simulink model "Simulink_File"  (R2021a)
settings: Solver=VariableStepAuto  StartTime=0.0  StopTime=10.0  RelTol=1e-3
undefined symbols (not defined in the file or in its folder): A, B, C, D, x0
libraries: vrlib x2, aerolibanimutils x1
settings Model: Creator=J44381  LastModifiedBy=vicen
settings SolverCC: AlgebraicLoopSolver=TrustRegion
settings DebuggingCC: SFMachineParentedDataDiag=warning

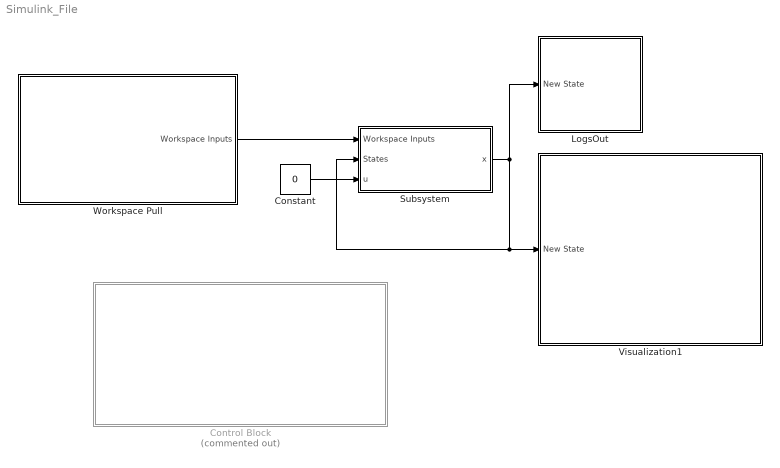
== system Simulink_File ==
  Constant : Constant  Value=0
  Control Block : Subsystem  Commented=on
  LogsOut : Subsystem
  Subsystem : Subsystem
  Visualization1 : Subsystem
  Workspace Pull : Subsystem
  wires:
  Workspace Pull/1("Workspace Inputs ") -> Subsystem/1("Workspace Inputs ")
  Subsystem/1(x) -> LogsOut/1(New State), Visualization1/1(New State), Subsystem/2(States)
  Constant/1 -> Subsystem/3(u)

== system Simulink_File/Control Block ==

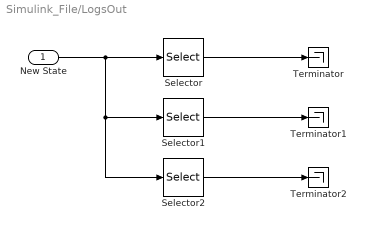
== system Simulink_File/LogsOut ==
  New State : Inport
  Selector : Selector  InputPortWidth=6  IndexOptions=Index vector (dialog)  Indices=1  OutputSizes=1
  Selector1 : Selector  InputPortWidth=6  IndexOptions=Index vector (dialog)  Indices=2  OutputSizes=1
  Selector2 : Selector  InputPortWidth=6  IndexOptions=Index vector (dialog)  Indices=3  OutputSizes=1
  Terminator : Terminator
  Terminator1 : Terminator
  Terminator2 : Terminator
  wires:
  Selector/1 -> Terminator/1
  Selector1/1 -> Terminator1/1
  Selector2/1 -> Terminator2/1
  New State/1 -> Selector2/1, Selector1/1, Selector/1

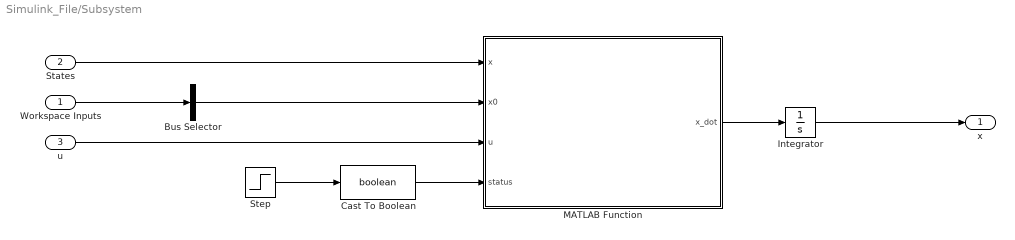
== system Simulink_File/Subsystem ==
  "Workspace Inputs " : Inport
  States : Inport  Port=2
  u : Inport  Port=3
  Bus Selector : BusSelector  OutputSignals=Initial States  OutputAsBus=on
  Cast To Boolean : DataTypeConversion  OutDataTypeStr=boolean
  Integrator : Integrator  InitialCondition=[x0.x;x0.theta1;x0.theta2;x0.x_dot;x0.theta1_dot;x0.theta2_dot]
  MATLAB Function : MATLAB Function  TreatAsAtomicUnit=on
  Step : Step  SampleTime=0
  x : Outport
  wires:
  MATLAB Function/1(x_dot) -> Integrator/1
  States/1 -> MATLAB Function/1(x)
  "Workspace Inputs "/1 -> Bus Selector/1
  u/1 -> MATLAB Function/3(u)
  Bus Selector/1 -> MATLAB Function/2(x0)
  Integrator/1 -> x/1
  Step/1 -> Cast To Boolean/1
  Cast To Boolean/1 -> MATLAB Function/4(status)

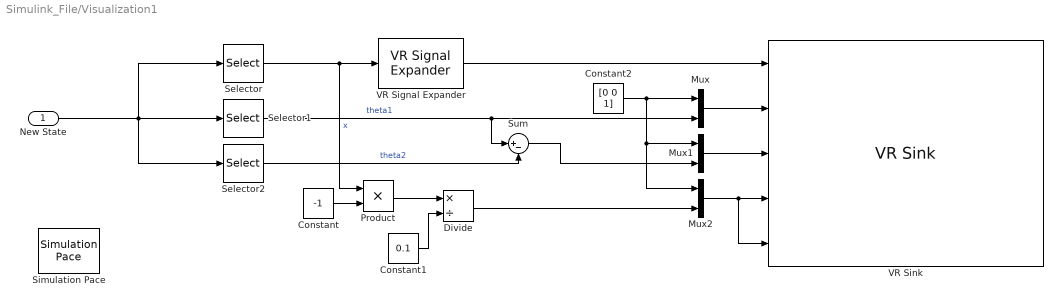
== system Simulink_File/Visualization1 ==
  New State : Inport
  Constant : Constant  Value=-1
  Constant1 : Constant  Value=0.1
  Constant2 : Constant  Value=[0 0 1]
  Divide : Product  Inputs=*/
  Mux : Mux  Inputs=2
  Mux1 : Mux  Inputs=2
  Mux2 : Mux  Inputs=2
  Product : Product
  Selector : Selector  InputPortWidth=6  IndexOptions=Index vector (dialog)  Indices=1  OutputSizes=1
  Selector1 : Selector  InputPortWidth=6  IndexOptions=Index vector (dialog)  Indices=2  OutputSizes=1
  Selector2 : Selector  InputPortWidth=6  IndexOptions=Index vector (dialog)  Indices=3  OutputSizes=1
  Simulation Pace : aerolibanimutils/Simulation Pace  SimulationPace=1  SleepMode=Auto  OutputPaceError=off  SampleTime=1/30
  Sum : Sum  Inputs=|+-
  VR Signal Expander : vrlib/VR Signal Expander  outwidth=3  outidx=[1]
  VR Sink : vrlib/VR Sink  InstantiateOnLoad=on  SampleTime=0.1  ViewEnable=on  RemoteChange=off  RemoteView=off  FieldsWritten=Cart.translation.3.1.1.double#Rotation1.rotation.4.1.1.double#Rotation2.rotation.4.1.1.double#Axis_Rotate.rotation.4.1.1.double#Axis_Rotate2.rotation.4.1.1.double  WorldFileName=Cart_Actual.WRL  AutoView=off  VideoDimensions=[]  AllowVariableSize=off
  wires:
  New State/1 -> Selector/1, Selector2/1, Selector1/1
  Selector/1 -> VR Signal Expander/1, Product/1  "x"
  Selector1/1 -> Sum/1, Mux/2  "theta1"
  Product/1 -> Divide/1
  Constant/1 -> Product/2
  Constant1/1 -> Divide/2
  Constant2/1 -> Mux1/1, Mux2/1, Mux/1
  Selector2/1 -> Sum/2  "theta2"
  Divide/1 -> Mux2/2
  Sum/1 -> Mux1/2
  VR Signal Expander/1 -> VR Sink/1
  Mux/1 -> VR Sink/2
  Mux1/1 -> VR Sink/3
  Mux2/1 -> VR Sink/4, VR Sink/5

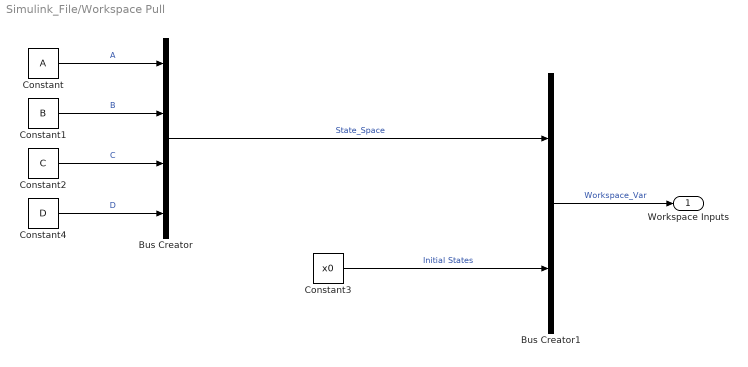
== system Simulink_File/Workspace Pull ==
  Bus Creator : BusCreator  Inputs=4
  Bus Creator1 : BusCreator  Inputs=2
  Constant : Constant  Value=A  VectorParams1D=off
  Constant1 : Constant  Value=B  VectorParams1D=off
  Constant2 : Constant  Value=C  VectorParams1D=off
  Constant3 : Constant  Value=x0  VectorParams1D=off  OutDataTypeStr=Bus: State_bus
  Constant4 : Constant  Value=D  VectorParams1D=off
  "Workspace Inputs " : Outport
  wires:
  Constant/1 -> Bus Creator/1  "A"
  Constant1/1 -> Bus Creator/2  "B"
  Constant2/1 -> Bus Creator/3  "C"
  Constant4/1 -> Bus Creator/4  "D"
  Bus Creator/1 -> Bus Creator1/1  "State_Space"
  Bus Creator1/1 -> "Workspace Inputs "/1  "Workspace_Var"
  Constant3/1 -> Bus Creator1/2  "Initial States"

== matlab function Simulink_File/Subsystem/MATLAB Function ==
  data: x input; x0 input; u input; x_dot output; status input
function x_dot  = Nonlinear_Dynamics(x,x0,u,status)
    if status == false
        x2 = x0.theta1;
        x3 = x0.theta2;
        x4 = x0.x_dot;
        x5 = x0.theta1_dot;
        x6 = x0.theta2_dot;
        u1 = u;
    else
        x2 = x(2);
        x3 = x(3);
        x4 = x(4);
        x5 = x(5);
        x6 = x(6);
        u1 = u;
    end
    % Insert Equations
    x_dot = double([
       x4;
       x5;
       x6;
       x5*((15*x5*sin(x2 - x3)*(cos(x3) - cos(x2 - x3)*cos(x2)))/(2*(25*cos(x2)^2 + 15*cos(x3)^2 + 33*cos(x2 - x3)^2 - 30*cos(x2 - x3)*cos(x2)*cos(x3) - 55)) + (5*x5*sin(x2)*(3*cos(x2 - x3)^2 - 5))/(2*(25*cos(x2)^2 + 15*cos(x3)^2 + 33*cos(x2 - x3)^2 - 30*cos(x2 - x3)*cos(x2)*cos(x3) - 55))) - x6*((9*x6*sin(x2 - x3)*(5*cos(x2) - 3*cos(x2 - x3)*cos(x3)))/(4*(25*cos(x2)^2 + 15*cos(x3)^2 + 33*cos(x2 - x3)^2 - 30*cos(x2 - x3)*cos(x2)*cos(x3) - 55)) - (9*x6*sin(x3)*(3*cos(x2 - x3)^2 - 5))/(4*(25*cos(x2)^2 + 15*cos(x3)^2 + 33*cos(x2 - x3)^2 - 30*cos(x2 - x3)*cos(x2)*cos(x3) - 55))) + (981*sin(x2)*(5*cos(x2) - 3*cos(x2 - x3)*cos(x3)))/(20*(25*cos(x2)^2 + 15*cos(x3)^2 + 33*cos(x2 - x3)^2 - 30*cos(x2 - x3)*cos(x2)*cos(x3) - 55)) + (2943*sin(x3)*(cos(x3) - cos(x2 - x3)*cos(x2)))/(20*(25*cos(x2)^2 + 15*cos(x3)^2 + 33*cos(x2 - x3)^2 - 30*cos(x2 - x3)*cos(x2)*cos(x3) - 55)) + (4*u1*(3*cos(x2 - x3)^2 - 5))/(25*cos(x2)^2 + 15*cos(x3)^2 + 33*cos(x2 - x3)^2 - 30*cos(x2 - x3)*cos(x2)*cos(x3) - 55);
       x5*((5*x5*sin(x2)*(5*cos(x2) - 3*cos(x2 - x3)*cos(x3)))/(25*cos(x2)^2 + 15*cos(x3)^2 + 33*cos(x2 - x3)^2 - 30*cos(x2 - x3)*cos(x2)*cos(x3) - 55) + (3*x5*sin(x2 - x3)*(11*cos(x2 - x3) - 5*cos(x2)*cos(x3)))/(25*cos(x2)^2 + 15*cos(x3)^2 + 33*cos(x2 - x3)^2 - 30*cos(x2 - x3)*cos(x2)*cos(x3) - 55)) + x6*((9*x6*sin(x3)*(5*cos(x2) - 3*cos(x2 - x3)*cos(x3)))/(2*(25*cos(x2)^2 + 15*cos(x3)^2 + 33*cos(x2 - x3)^2 - 30*cos(x2 - x3)*cos(x2)*cos(x3) - 55)) - (9*x6*sin(x2 - x3)*(3*cos(x3)^2 - 11))/(2*(25*cos(x2)^2 + 15*cos(x3)^2 + 33*cos(x2 - x3)^2 - 30*cos(x2 - x3)*cos(x2)*cos(x3) - 55))) + (2943*sin(x3)*(11*cos(x2 - x3) - 5*cos(x2)*cos(x3)))/(50*(25*cos(x2)^2 + 15*cos(x3)^2 + 33*cos(x2 - x3)^2 - 30*cos(x2 - x3)*cos(x2)*cos(x3) - 55)) + (981*sin(x2)*(3*cos(x3)^2 - 11))/(10*(25*cos(x2)^2 + 15*cos(x3)^2 + 33*cos(x2 - x3)^2 - 30*cos(x2 - x3)*cos(x2)*cos(x3) - 55)) + (8*u1*(5*cos(x2) - 3*cos(x2 - x3)*cos(x3)))/(25*cos(x2)^2 + 15*cos(x3)^2 + 33*cos(x2 - x3)^2 - 30*cos(x2 - x3)*cos(x2)*cos(x3) - 55);
       x6*((15*x6*sin(x3)*(cos(x3) - cos(x2 - x3)*cos(x2)))/(25*cos(x2)^2 + 15*cos(x3)^2 + 33*cos(x2 - x3)^2 - 30*cos(x2 - x3)*cos(x2)*cos(x3) - 55) - (3*x6*sin(x2 - x3)*(11*cos(x2 - x3) - 5*cos(x2)*cos(x3)))/(25*cos(x2)^2 + 15*cos(x3)^2 + 33*cos(x2 - x3)^2 - 30*cos(x2 - x3)*cos(x2)*cos(x3) - 55)) + x5*((50*x5*sin(x2)*(cos(x3) - cos(x2 - x3)*cos(x2)))/(3*(25*cos(x2)^2 + 15*cos(x3)^2 + 33*cos(x2 - x3)^2 - 30*cos(x2 - x3)*cos(x2)*cos(x3) - 55)) + (10*x5*sin(x2 - x3)*(5*cos(x2)^2 - 11))/(3*(25*cos(x2)^2 + 15*cos(x3)^2 + 33*cos(x2 - x3)^2 - 30*cos(x2 - x3)*cos(x2)*cos(x3) - 55))) + (327*sin(x2)*(11*cos(x2 - x3) - 5*cos(x2)*cos(x3)))/(5*(25*cos(x2)^2 + 15*cos(x3)^2 + 33*cos(x2 - x3)^2 - 30*cos(x2 - x3)*cos(x2)*cos(x3) - 55)) + (327*sin(x3)*(5*cos(x2)^2 - 11))/(5*(25*cos(x2)^2 + 15*cos(x3)^2 + 33*cos(x2 - x3)^2 - 30*cos(x2 - x3)*cos(x2)*cos(x3) - 55)) + (80*u1*(cos(x3) - cos(x2 - x3)*cos(x2)))/(3*(25*cos(x2)^2 + 15*cos(x3)^2 + 33*cos(x2 - x3)^2 - 30*cos(x2 - x3)*cos(x2)*cos(x3) - 55))]);
    
end
